simulink model "exampleModel_bus_axi_w_4ptavg"  (R2017b)
settings: Solver=VariableStepAuto  StartTime=0.0  StopTime=10e-5  RelTol=1e-3
PreLoadFcn:
  | setup
values from neighbouring files (symbols this model uses):
  axiClk = 156.25e6    (= 156250000)    [setup.m]    (also in setup_exampleModel_bus_axi_simulink.m; setup_exampleModel_bus_axi_simulink_lcls2.m; setup_lcls2_pcav.m; sysgen_signal.m)
  cav1p1_addr = 204    [setup_exampleModel_bus_axi_simulink.m]    (also in setup_exampleModel_bus_axi_simulink_lcls2.m; setup_lcls2_pcav.m; sysgen_signal.m)
  cav1p2_addr = cav1p1_addr * 2    (= 408)    [setup_exampleModel_bus_axi_simulink.m]    (also in setup_exampleModel_bus_axi_simulink_lcls2.m; setup_lcls2_pcav.m; sysgen_signal.m)
  cav2p1_addr = cav1p1_addr * 3    (= 612)    [setup_exampleModel_bus_axi_simulink.m]    (also in setup_exampleModel_bus_axi_simulink_lcls2.m; setup_lcls2_pcav.m; sysgen_signal.m)
  cav2p2_addr = cav1p1_addr * 4    (= 816)    [setup_exampleModel_bus_axi_simulink.m]    (also in setup_exampleModel_bus_axi_simulink_lcls2.m; setup_lcls2_pcav.m; sysgen_signal.m)
  Fadc = Fs/interleavedChannels    (= 29750000)    [setup.m]    (also in setup_exampleModel_bus_axi_simulink.m = 357000000; setup_exampleModel_bus_axi_simulink_lcls2.m = 351000000; setup_lcls2_pcav.m = 357000000; sysgen_signal.m = 357000000)
  fir_lpf = fir1(15, w_lpf)    [setup_exampleModel_bus_axi_simulink.m]    (also in setup_exampleModel_bus_axi_simulink_lcls2.m; setup_lcls2_pcav.m)
  Fproc = 204e6    (= 204000000)    [setup_exampleModel_bus_axi_simulink.m]    (also in setup_exampleModel_bus_axi_simulink_lcls2.m = 200571400; setup_lcls2_pcav.m; sysgen_signal.m)
  Fsig = Fproc/12    (= 17000000)    [setup_exampleModel_bus_axi_simulink.m]    (also in setup_exampleModel_bus_axi_simulink_lcls2.m = 16714283.3333; setup_lcls2_pcav.m)
  Tadc = 1/fadc    (= 2.80112044818e-09)    [cavity_signal.m]    (also in setup_exampleModel_bus_axi_simulink.m; setup_exampleModel_bus_axi_simulink_lcls2.m = 2.849002849e-09; setup_lcls2_pcav.m; setup_pcav_simulink.m)
undefined symbols (not defined in the file or in its folder): AXI4, Lite
libraries: xbsIndex_r4 x2870, llrf_lib x10, simulink x3
(part 2 of 15)

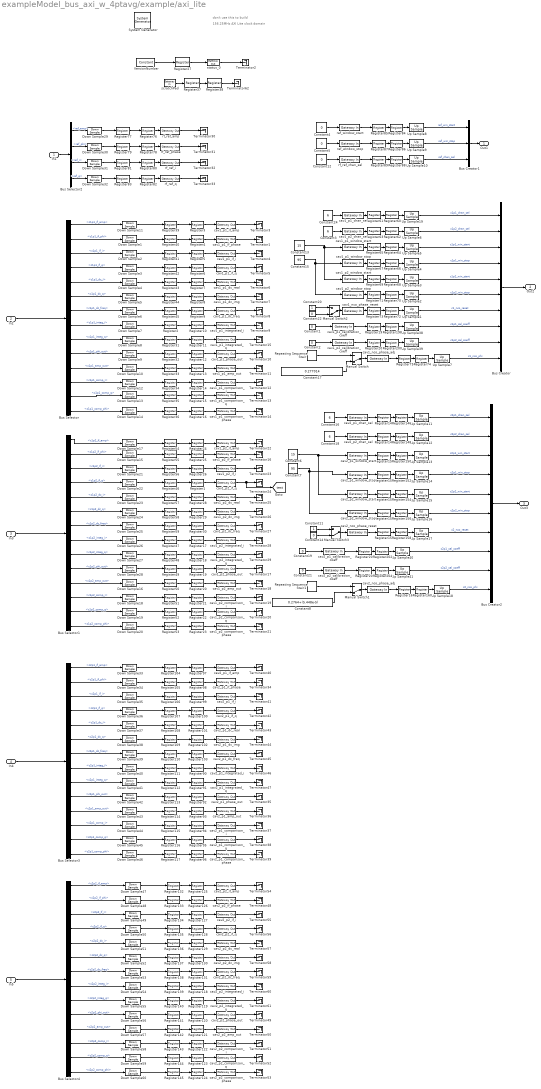
== system exampleModel_bus_axi_w_4ptavg/example/axi_lite ==
  note: don't use this to build
  note: 156.25MHz AXI Lite clock domain
  In1 : Inport
  In2 : Inport  Port=2
  In3 : Inport  Port=3
  In4 : Inport  Port=4
  In5 : Inport  Port=5
  " System Generator" : xbsIndex_r4/ System Generator  Tag=genX  xilinxfamily=kintexu  part=xcku040  speed=-2-e  package=ffva1156  synthesis_tool=Vivado  clock_wrapper=Clock Enables  directory=./netlist  proj_type=Vivado  Synth_file=Vivado Synthesis Defaults  Impl_file=Vivado Implementation Defaults  testbench=off  simulink_period=1/axiClk  sysclk_period=1e9/axiClk  dcm_input_clock_period=10  incr_netlist=off  trim_vbits=Everywhere in SubSystem  dbl_ovrd=According to Block Masks  core_generation=According to Block Masks  run_coregen=off  deprecated_control=off  eval_field=0  block_type=sysgen
  Bus Creator : BusCreator  Inputs=10
  Bus Creator1 : BusCreator  Inputs=3
  Bus Creator2 : BusCreator  Inputs=10
  Bus Selector : BusSelector  OutputSignals=c1p1_if_amp,c1p1_if_phi,c1p1_if_i,c1p1_if_q,c1p1_dc_i,c1p1_dc_q,c1p1_dc_freq,c1p1_integ_i,c1p1_integ_q,c1p1_phi_out,c1p1_amp_out,c1p1_comp_i,c1p1_comp_q,c1p1_comp_phi
  Bus Selector1 : BusSelector  OutputSignals=c1p2_if_amp,c1p2_if_phi,c1p2_if_i,c1p2_if_q,c1p2_dc_i,c1p2_dc_q,c1p2_dc_freq,c1p2_integ_i,c1p2_integ_q,c1p2_phi_out,c1p2_amp_out,c1p2_comp_i,c1p2_comp_q,c1p2_comp_phi
  Bus Selector2 : BusSelector  OutputSignals=ref_amp,ref_phi,ref_i,ref_q
  Bus Selector3 : BusSelector  OutputSignals=c2p1_if_amp,c2p1_if_phi,c2p1_if_i,c2p1_if_q,c2p1_dc_i,c2p1_dc_q,c2p1_dc_freq,c2p1_integ_i,c2p1_integ_q,c2p1_phi_out,c2p1_amp_out,c2p1_comp_i,c2p1_comp_q,c2p1_comp_phi
  Bus Selector4 : BusSelector  OutputSignals=c2p2_if_amp,c2p2_if_phi,c2p2_if_i,c2p2_if_q,c2p2_dc_i,c2p2_dc_q,c2p2_dc_freq,c2p2_integ_i,c2p2_integ_q,c2p2_phi_out,c2p2_amp_out,c2p2_comp_i,c2p2_comp_q,c2p2_comp_phi
  Constant{1..2,4..5,12,14,19,21..22} (9 alike) : Constant  Value=0  SampleTime=8/axiClk
  Constant11 : Constant  SampleTime=8/axiClk
  Constant13 : Constant  Value=15  SampleTime=8/axiClk
  Constant15 : Constant  Value=95  SampleTime=8/axiClk
  Constant{3,16,18,24} (4 alike) : Constant  Value=6  SampleTime=8/axiClk
  Constant17 : Constant  Value=0.277014  VectorParams1D=off  SampleTime=8/axiClk
  Constant20 : Constant  SampleTime=8/axiClk
  Constant6 : Constant  Value=15  SampleTime=8/axiClk
  Constant7 : Constant  Value=95  SampleTime=8/axiClk
  Constant8 : Constant  Value=0.2764+(5.448e-5)  VectorParams1D=off  SampleTime=8/axiClk
  Down Sample{1..60} (60 alike) : xbsIndex_r4/Down Sample  sample_ratio=8  sample_phase="Last Value of Frame  (most efficient)"  en=off  rst=off  latency=1  dbl_ovrd=off  block_type=dsamp
  Manual Switch{,1..3} (4 alike) : ManualSwitch  CurrentSetting=0
  Register{1..65,68..69,72..161,198..205} (165 alike) : xbsIndex_r4/Register  init=0  rst=off  en=off  dbl_ovrd=off  block_type=register
  Register{66..67,70..71} (4 alike) : xbsIndex_r4/Register  init=100  rst=off  en=off  dbl_ovrd=off  block_type=register
  Repeating Sequence Stair : simulink/Sources/Repeating Sequence Stair  OutValues=[0 (30/360) (45/360) (60/360) (75/360) (90/360) (8.2941/360)]  tsamp=0.5e-6  OutMin=[]  OutMax=[]  OutDataTypeStr=double  OutputDataTypeScalingMode=double  OutDataType=fixdt(0,8)  ConRadixGroup=Best Precision: Vector-wise  OutScaling=2^-12
  Repeating Sequence Stair1 : simulink/Sources/Repeating Sequence Stair  OutValues=[0 (30/360) (45/360) (60/360) (75/360) (90/360) (8.2941/360)]  tsamp=0.5e-6  OutMin=[]  OutMax=[]  OutDataTypeStr=double  OutputDataTypeScalingMode=double  OutDataType=fixdt(0,8)  ConRadixGroup=Best Precision: Vector-wise  OutScaling=2^-12
  Terminator{1..62} (62 alike) : Terminator
  Up Sample{1..19,38..41} (23 alike) : xbsIndex_r4/Up Sample  sample_ratio=8  copy_samples=on  en=off  latency=1  dbl_ovrd=off  block_type=usamp
  VersionNumber : xbsIndex_r4/Constant  const=7162020  gui_display_data_type=Fixed-point  arith_type=Unsigned  n_bits=32  bin_pt=0  preci_type=Single  exp_width=8  frac_width=24  explicit_period=on  period=8/axiClk  equ=P=C  opselect=C  inp2=PCIN>>17  opr=+  inp1=P  carry=CIN  dbl_ovrd=off  block_type=constant
  cav1_nco_phase_adj : xbsIndex_r4/Gateway In  gui_display_data_type=Fixed-point  arith_type=Unsigned  n_bits=32  bin_pt=32  preci_type=Single  exp_width=8  frac_width=24  rows=1  columns=1  quantization="Round  (unbiased: +/- Inf)"  overflow=Saturate  period=8/axiClk  UseAsADC=off  ADCChannel='1'  interface=AXI4-Lite  automatic_assignment=off  address_offset=cav1p1_addr+hex2dec('4C')  intf_name=''  intf_description=''  default_value=0  timing_constraint=None  locs_specified=off  LOCs={}  io_standard={}  inherit_from_input=off  hdl_port=on  dbl_ovrd=off  block_type=gatewayin
  cav1_nco_phase_reset : xbsIndex_r4/Gateway In  gui_display_data_type=Fixed-point  arith_type=Unsigned  n_bits=1  bin_pt=0  preci_type=Single  exp_width=8  frac_width=24  rows=1  columns=1  quantization="Round  (unbiased: +/- Inf)"  overflow=Saturate  period=8/axiClk  UseAsADC=off  ADCChannel='1'  interface=AXI4-Lite  automatic_assignment=off  address_offset=cav1p1_addr+hex2dec('50')  intf_name=''  intf_description=''  default_value=0  timing_constraint=None  locs_specified=off  LOCs={}  io_standard={}  inherit_from_input=off  hdl_port=on  dbl_ovrd=off  block_type=gatewayin
  cav1_p1_amp_out : xbsIndex_r4/Gateway Out  inherit_from_input=off  hdl_port=on  rows=1  columns=1  UseAsDAC=off  DACChannel='1'  interface=AXI4-Lite  automatic_assignment=off  address_offset=cav1p1_addr+hex2dec('34')  intf_name=''  intf_description=''  timing_constraint=None  locs_specified=off  LOCs={}  io_standard={}  block_type=gatewayout
  cav1_p1_calibration_coeff : xbsIndex_r4/Gateway In  gui_display_data_type=Fixed-point  arith_type=Unsigned  n_bits=18  bin_pt=17  preci_type=Single  exp_width=8  frac_width=24  rows=1  columns=1  quantization="Round  (unbiased: +/- Inf)"  overflow=Saturate  period=8/axiClk  UseAsADC=off  ADCChannel='1'  interface=AXI4-Lite  automatic_assignment=off  address_offset=cav1p1_addr+hex2dec('48')  intf_name=''  intf_description=''  default_value=0  timing_constraint=None  locs_specified=off  LOCs={}  io_standard={}  inherit_from_input=off  hdl_port=on  dbl_ovrd=off  block_type=gatewayin
  cav1_p1_chan_sel : xbsIndex_r4/Gateway In  gui_display_data_type=Fixed-point  arith_type=Unsigned  n_bits=4  bin_pt=0  preci_type=Single  exp_width=8  frac_width=24  rows=1  columns=1  quantization="Round  (unbiased: +/- Inf)"  overflow=Saturate  period=8/axiClk  UseAsADC=off  ADCChannel='1'  interface=AXI4-Lite  automatic_assignment=off  address_offset=cav1p1_addr+hex2dec('10')  intf_name=''  intf_description=''  default_value=0  timing_constraint=None  locs_specified=off  LOCs={}  io_standard={}  inherit_from_input=off  hdl_port=on  dbl_ovrd=off  block_type=gatewayin
  cav1_p1_comparison_i : xbsIndex_r4/Gateway Out  inherit_from_input=off  hdl_port=on  rows=1  columns=1  UseAsDAC=off  DACChannel='1'  interface=AXI4-Lite  automatic_assignment=off  address_offset=cav1p1_addr+hex2dec('38')  intf_name=''  intf_description=''  timing_constraint=None  locs_specified=off  LOCs={}  io_standard={}  block_type=gatewayout
  cav1_p1_comparison_phase : xbsIndex_r4/Gateway Out  inherit_from_input=off  hdl_port=on  rows=1  columns=1  UseAsDAC=off  DACChannel='1'  interface=AXI4-Lite  automatic_assignment=off  address_offset=cav1p1_addr+hex2dec('40')  intf_name=''  intf_description=''  timing_constraint=None  locs_specified=off  LOCs={}  io_standard={}  block_type=gatewayout
  cav1_p1_comparison_q : xbsIndex_r4/Gateway Out  inherit_from_input=off  hdl_port=on  rows=1  columns=1  UseAsDAC=off  DACChannel='1'  interface=AXI4-Lite  automatic_assignment=off  address_offset=cav1p1_addr+hex2dec('3C')  intf_name=''  intf_description=''  timing_constraint=None  locs_specified=off  LOCs={}  io_standard={}  block_type=gatewayout
  cav1_p1_dc_freq : xbsIndex_r4/Gateway Out  inherit_from_input=off  hdl_port=on  rows=1  columns=1  UseAsDAC=off  DACChannel='1'  interface=AXI4-Lite  automatic_assignment=off  address_offset=cav1p1_addr+hex2dec('24')  intf_name=''  intf_description=''  timing_constraint=None  locs_specified=off  LOCs={}  io_standard={}  block_type=gatewayout
  cav1_p1_dc_img : xbsIndex_r4/Gateway Out  inherit_from_input=off  hdl_port=on  rows=1  columns=1  UseAsDAC=off  DACChannel='1'  interface=AXI4-Lite  automatic_assignment=off  address_offset=cav1p1_addr+hex2dec('18')  intf_name=''  intf_description=''  timing_constraint=None  locs_specified=off  LOCs={}  io_standard={}  block_type=gatewayout
  cav1_p1_dc_real : xbsIndex_r4/Gateway Out  inherit_from_input=off  hdl_port=on  rows=1  columns=1  UseAsDAC=off  DACChannel='1'  interface=AXI4-Lite  automatic_assignment=off  address_offset=cav1p1_addr+hex2dec('14')  intf_name=''  intf_description=''  timing_constraint=None  locs_specified=off  LOCs={}  io_standard={}  block_type=gatewayout
  cav1_p1_if_amp : xbsIndex_r4/Gateway Out  inherit_from_input=off  hdl_port=on  rows=1  columns=1  UseAsDAC=off  DACChannel='1'  interface=AXI4-Lite  automatic_assignment=off  address_offset=cav1p1_addr+hex2dec('00')  intf_name=''  intf_description=''  timing_constraint=None  locs_specified=off  LOCs={}  io_standard={}  block_type=gatewayout
  cav1_p1_if_i : xbsIndex_r4/Gateway Out  inherit_from_input=off  hdl_port=on  rows=1  columns=1  UseAsDAC=off  DACChannel='1'  interface=AXI4-Lite  automatic_assignment=off  address_offset=cav1p1_addr+hex2dec('8')  intf_name=''  intf_description=''  timing_constraint=None  locs_specified=off  LOCs={}  io_standard={}  block_type=gatewayout
  cav1_p1_if_phase : xbsIndex_r4/Gateway Out  inherit_from_input=off  hdl_port=on  rows=1  columns=1  UseAsDAC=off  DACChannel='1'  interface=AXI4-Lite  automatic_assignment=off  address_offset=cav1p1_addr+hex2dec('4')  intf_name=''  intf_description=''  timing_constraint=None  locs_specified=off  LOCs={}  io_standard={}  block_type=gatewayout
  cav1_p1_if_q : xbsIndex_r4/Gateway Out  inherit_from_input=off  hdl_port=on  rows=1  columns=1  UseAsDAC=off  DACChannel='1'  interface=AXI4-Lite  automatic_assignment=off  address_offset=cav1p1_addr+hex2dec('c')  intf_name=''  intf_description=''  timing_constraint=None  locs_specified=off  LOCs={}  io_standard={}  block_type=gatewayout
  cav1_p1_integrated_i : xbsIndex_r4/Gateway Out  inherit_from_input=off  hdl_port=on  rows=1  columns=1  UseAsDAC=off  DACChannel='1'  interface=AXI4-Lite  automatic_assignment=off  address_offset=cav1p1_addr+hex2dec('28')  intf_name=''  intf_description=''  timing_constraint=None  locs_specified=off  LOCs={}  io_standard={}  block_type=gatewayout
  cav1_p1_integrated_q : xbsIndex_r4/Gateway Out  inherit_from_input=off  hdl_port=on  rows=1  columns=1  UseAsDAC=off  DACChannel='1'  interface=AXI4-Lite  automatic_assignment=off  address_offset=cav1p1_addr+hex2dec('2c')  intf_name=''  intf_description=''  timing_constraint=None  locs_specified=off  LOCs={}  io_standard={}  block_type=gatewayout
  cav1_p1_phase_out : xbsIndex_r4/Gateway Out  inherit_from_input=off  hdl_port=on  rows=1  columns=1  UseAsDAC=off  DACChannel='1'  interface=AXI4-Lite  automatic_assignment=off  address_offset=cav1p1_addr+hex2dec('30')  intf_name=''  intf_description=''  timing_constraint=None  locs_specified=off  LOCs={}  io_standard={}  block_type=gatewayout
  cav1_p1_window_start : xbsIndex_r4/Gateway In  gui_display_data_type=Fixed-point  arith_type=Unsigned  n_bits=16  bin_pt=0  preci_type=Single  exp_width=8  frac_width=24  rows=1  columns=1  quantization="Round  (unbiased: +/- Inf)"  overflow=Saturate  period=8/axiClk  UseAsADC=off  ADCChannel='1'  interface=AXI4-Lite  automatic_assignment=off  address_offset=cav1p1_addr+hex2dec('1C')  intf_name=''  intf_description=''  default_value=0  timing_constraint=None  locs_specified=off  LOCs={}  io_standard={}  inherit_from_input=off  hdl_port=on  dbl_ovrd=off  block_type=gatewayin
  cav1_p1_window_stop : xbsIndex_r4/Gateway In  gui_display_data_type=Fixed-point  arith_type=Unsigned  n_bits=16  bin_pt=0  preci_type=Single  exp_width=8  frac_width=24  rows=1  columns=1  quantization="Round  (unbiased: +/- Inf)"  overflow=Saturate  period=8/axiClk  UseAsADC=off  ADCChannel='1'  interface=AXI4-Lite  automatic_assignment=off  address_offset=cav1p1_addr+hex2dec('20')  intf_name=''  intf_description=''  default_value=100  timing_constraint=None  locs_specified=off  LOCs={}  io_standard={}  inherit_from_input=off  hdl_port=on  dbl_ovrd=off  block_type=gatewayin
  cav1_p2_amp_out : xbsIndex_r4/Gateway Out  inherit_from_input=off  hdl_port=on  rows=1  columns=1  UseAsDAC=off  DACChannel='1'  interface=AXI4-Lite  automatic_assignment=off  address_offset=cav1p2_addr+hex2dec('34')  intf_name=''  intf_description=''  timing_constraint=None  locs_specified=off  LOCs={}  io_standard={}  block_type=gatewayout
  cav1_p2_calibration_coeff : xbsIndex_r4/Gateway In  gui_display_data_type=Fixed-point  arith_type=Unsigned  n_bits=18  bin_pt=17  preci_type=Single  exp_width=8  frac_width=24  rows=1  columns=1  quantization="Round  (unbiased: +/- Inf)"  overflow=Saturate  period=8/axiClk  UseAsADC=off  ADCChannel='1'  interface=AXI4-Lite  automatic_assignment=off  address_offset=cav1p2_addr+hex2dec('48')  intf_name=''  intf_description=''  default_value=0  timing_constraint=None  locs_specified=off  LOCs={}  io_standard={}  inherit_from_input=off  hdl_port=on  dbl_ovrd=off  block_type=gatewayin
  cav1_p2_chan_sel : xbsIndex_r4/Gateway In  gui_display_data_type=Fixed-point  arith_type=Unsigned  n_bits=4  bin_pt=0  preci_type=Single  exp_width=8  frac_width=24  rows=1  columns=1  quantization="Round  (unbiased: +/- Inf)"  overflow=Saturate  period=8/axiClk  UseAsADC=off  ADCChannel='1'  interface=AXI4-Lite  automatic_assignment=off  address_offset=cav1p2_addr+hex2dec('10')  intf_name=''  intf_description=''  default_value=0  timing_constraint=None  locs_specified=off  LOCs={}  io_standard={}  inherit_from_input=off  hdl_port=on  dbl_ovrd=off  block_type=gatewayin
  cav1_p2_comparison_i : xbsIndex_r4/Gateway Out  inherit_from_input=off  hdl_port=on  rows=1  columns=1  UseAsDAC=off  DACChannel='1'  interface=AXI4-Lite  automatic_assignment=off  address_offset=cav1p2_addr+hex2dec('38')  intf_name=''  intf_description=''  timing_constraint=None  locs_specified=off  LOCs={}  io_standard={}  block_type=gatewayout
  cav1_p2_comparison_phase : xbsIndex_r4/Gateway Out  inherit_from_input=off  hdl_port=on  rows=1  columns=1  UseAsDAC=off  DACChannel='1'  interface=AXI4-Lite  automatic_assignment=off  address_offset=cav1p2_addr+hex2dec('40')  intf_name=''  intf_description=''  timing_constraint=None  locs_specified=off  LOCs={}  io_standard={}  block_type=gatewayout
  cav1_p2_comparison_q : xbsIndex_r4/Gateway Out  inherit_from_input=off  hdl_port=on  rows=1  columns=1  UseAsDAC=off  DACChannel='1'  interface=AXI4-Lite  automatic_assignment=off  address_offset=cav1p2_addr+hex2dec('3c')  intf_name=''  intf_description=''  timing_constraint=None  locs_specified=off  LOCs={}  io_standard={}  block_type=gatewayout
  cav1_p2_dc_freq : xbsIndex_r4/Gateway Out  inherit_from_input=off  hdl_port=on  rows=1  columns=1  UseAsDAC=off  DACChannel='1'  interface=AXI4-Lite  automatic_assignment=off  address_offset=cav1p2_addr+hex2dec('24')  intf_name=''  intf_description=''  timing_constraint=None  locs_specified=off  LOCs={}  io_standard={}  block_type=gatewayout
  cav1_p2_dc_img : xbsIndex_r4/Gateway Out  inherit_from_input=off  hdl_port=on  rows=1  columns=1  UseAsDAC=off  DACChannel='1'  interface=AXI4-Lite  automatic_assignment=off  address_offset=cav1p2_addr+hex2dec('18')  intf_name=''  intf_description=''  timing_constraint=None  locs_specified=off  LOCs={}  io_standard={}  block_type=gatewayout
  cav1_p2_dc_real : xbsIndex_r4/Gateway Out  inherit_from_input=off  hdl_port=on  rows=1  columns=1  UseAsDAC=off  DACChannel='1'  interface=AXI4-Lite  automatic_assignment=off  address_offset=cav1p2_addr+hex2dec('14')  intf_name=''  intf_description=''  timing_constraint=None  locs_specified=off  LOCs={}  io_standard={}  block_type=gatewayout
  cav1_p2_if_amp : xbsIndex_r4/Gateway Out  inherit_from_input=off  hdl_port=on  rows=1  columns=1  UseAsDAC=off  DACChannel='1'  interface=AXI4-Lite  automatic_assignment=off  address_offset=cav1p2_addr+hex2dec('00')  intf_name=''  intf_description=''  timing_constraint=None  locs_specified=off  LOCs={}  io_standard={}  block_type=gatewayout
  "cav1_p2_if_i " : xbsIndex_r4/Gateway Out  inherit_from_input=off  hdl_port=on  rows=1  columns=1  UseAsDAC=off  DACChannel='1'  interface=AXI4-Lite  automatic_assignment=off  address_offset=cav1p2_addr+hex2dec('08')  intf_name=''  intf_description=''  timing_constraint=None  locs_specified=off  LOCs={}  io_standard={}  block_type=gatewayout
  cav1_p2_if_phase : xbsIndex_r4/Gateway Out  inherit_from_input=off  hdl_port=on  rows=1  columns=1  UseAsDAC=off  DACChannel='1'  interface=AXI4-Lite  automatic_assignment=off  address_offset=cav1p2_addr+hex2dec('04')  intf_name=''  intf_description=''  timing_constraint=None  locs_specified=off  LOCs={}  io_standard={}  block_type=gatewayout
  cav1_p2_if_q : xbsIndex_r4/Gateway Out  inherit_from_input=off  hdl_port=on  rows=1  columns=1  UseAsDAC=off  DACChannel='1'  interface=AXI4-Lite  automatic_assignment=off  address_offset=cav1p2_addr+hex2dec('0C')  intf_name=''  intf_description=''  timing_constraint=None  locs_specified=off  LOCs={}  io_standard={}  block_type=gatewayout
  cav1_p2_integrated_i : xbsIndex_r4/Gateway Out  inherit_from_input=off  hdl_port=on  rows=1  columns=1  UseAsDAC=off  DACChannel='1'  interface=AXI4-Lite  automatic_assignment=off  address_offset=cav1p2_addr+hex2dec('28')  intf_name=''  intf_description=''  timing_constraint=None  locs_specified=off  LOCs={}  io_standard={}  block_type=gatewayout
  cav1_p2_integrated_q : xbsIndex_r4/Gateway Out  inherit_from_input=off  hdl_port=on  rows=1  columns=1  UseAsDAC=off  DACChannel='1'  interface=AXI4-Lite  automatic_assignment=off  address_offset=cav1p2_addr+hex2dec('2c')  intf_name=''  intf_description=''  timing_constraint=None  locs_specified=off  LOCs={}  io_standard={}  block_type=gatewayout
  cav1_p2_phase_out : xbsIndex_r4/Gateway Out  inherit_from_input=off  hdl_port=on  rows=1  columns=1  UseAsDAC=off  DACChannel='1'  interface=AXI4-Lite  automatic_assignment=off  address_offset=cav1p2_addr+hex2dec('30')  intf_name=''  intf_description=''  timing_constraint=None  locs_specified=off  LOCs={}  io_standard={}  block_type=gatewayout
  cav1_p2_window_start : xbsIndex_r4/Gateway In  gui_display_data_type=Fixed-point  arith_type=Unsigned  n_bits=16  bin_pt=0  preci_type=Single  exp_width=8  frac_width=24  rows=1  columns=1  quantization="Round  (unbiased: +/- Inf)"  overflow=Saturate  period=8/axiClk  UseAsADC=off  ADCChannel='1'  interface=AXI4-Lite  automatic_assignment=off  address_offset=cav1p2_addr+hex2dec('1c')  intf_name=''  intf_description=''  default_value=0  timing_constraint=None  locs_specified=off  LOCs={}  io_standard={}  inherit_from_input=off  hdl_port=on  dbl_ovrd=off  block_type=gatewayin
  cav1_p2_window_stop : xbsIndex_r4/Gateway In  gui_display_data_type=Fixed-point  arith_type=Unsigned  n_bits=16  bin_pt=0  preci_type=Single  exp_width=8  frac_width=24  rows=1  columns=1  quantization="Round  (unbiased: +/- Inf)"  overflow=Saturate  period=8/axiClk  UseAsADC=off  ADCChannel='1'  interface=AXI4-Lite  automatic_assignment=off  address_offset=cav1p2_addr+hex2dec('20')  intf_name=''  intf_description=''  default_value=100  timing_constraint=None  locs_specified=off  LOCs={}  io_standard={}  inherit_from_input=off  hdl_port=on  dbl_ovrd=off  block_type=gatewayin
  cav2_nco_phase_adj : xbsIndex_r4/Gateway In  gui_display_data_type=Fixed-point  arith_type=Unsigned  n_bits=32  bin_pt=32  preci_type=Single  exp_width=8  frac_width=24  rows=1  columns=1  quantization="Round  (unbiased: +/- Inf)"  overflow=Saturate  period=8/axiClk  UseAsADC=off  ADCChannel='1'  interface=AXI4-Lite  automatic_assignment=off  address_offset=cav2p1_addr+hex2dec('4c')  intf_name=''  intf_description=''  default_value=0  timing_constraint=None  locs_specified=off  LOCs={}  io_standard={}  inherit_from_input=off  hdl_port=on  dbl_ovrd=off  block_type=gatewayin
  cav2_nco_phase_reset : xbsIndex_r4/Gateway In  gui_display_data_type=Fixed-point  arith_type=Unsigned  n_bits=1  bin_pt=0  preci_type=Single  exp_width=8  frac_width=24  rows=1  columns=1  quantization="Round  (unbiased: +/- Inf)"  overflow=Saturate  period=8/axiClk  UseAsADC=off  ADCChannel='1'  interface=AXI4-Lite  automatic_assignment=off  address_offset=cav2p1_addr+hex2dec('50')  intf_name=''  intf_description=''  default_value=0  timing_constraint=None  locs_specified=off  LOCs={}  io_standard={}  inherit_from_input=off  hdl_port=on  dbl_ovrd=off  block_type=gatewayin
  cav2_p1_amp_out : xbsIndex_r4/Gateway Out  inherit_from_input=off  hdl_port=on  rows=1  columns=1  UseAsDAC=off  DACChannel='1'  interface=AXI4-Lite  automatic_assignment=off  address_offset=cav2p1_addr+hex2dec('34')  intf_name=''  intf_description=''  timing_constraint=None  locs_specified=off  LOCs={}  io_standard={}  block_type=gatewayout
  cav2_p1_calibration_coeff : xbsIndex_r4/Gateway In  gui_display_data_type=Fixed-point  arith_type=Unsigned  n_bits=18  bin_pt=17  preci_type=Single  exp_width=8  frac_width=24  rows=1  columns=1  quantization="Round  (unbiased: +/- Inf)"  overflow=Saturate  period=8/axiClk  UseAsADC=off  ADCChannel='1'  interface=AXI4-Lite  automatic_assignment=off  address_offset=cav2p1_addr+hex2dec('48')  intf_name=''  intf_description=''  default_value=0  timing_constraint=None  locs_specified=off  LOCs={}  io_standard={}  inherit_from_input=off  hdl_port=on  dbl_ovrd=off  block_type=gatewayin
  cav2_p1_chan_sel : xbsIndex_r4/Gateway In  gui_display_data_type=Fixed-point  arith_type=Unsigned  n_bits=4  bin_pt=0  preci_type=Single  exp_width=8  frac_width=24  rows=1  columns=1  quantization="Round  (unbiased: +/- Inf)"  overflow=Saturate  period=8/axiClk  UseAsADC=off  ADCChannel='1'  interface=AXI4-Lite  automatic_assignment=off  address_offset=cav2p1_addr+hex2dec('10')  intf_name=''  intf_description=''  default_value=0  timing_constraint=None  locs_specified=off  LOCs={}  io_standard={}  inherit_from_input=off  hdl_port=on  dbl_ovrd=off  block_type=gatewayin
  cav2_p1_comparison_i : xbsIndex_r4/Gateway Out  inherit_from_input=off  hdl_port=on  rows=1  columns=1  UseAsDAC=off  DACChannel='1'  interface=AXI4-Lite  automatic_assignment=off  address_offset=cav2p1_addr+hex2dec('38')  intf_name=''  intf_description=''  timing_constraint=None  locs_specified=off  LOCs={}  io_standard={}  block_type=gatewayout
  cav2_p1_comparison_phase : xbsIndex_r4/Gateway Out  inherit_from_input=off  hdl_port=on  rows=1  columns=1  UseAsDAC=off  DACChannel='1'  interface=AXI4-Lite  automatic_assignment=off  address_offset=cav2p1_addr+hex2dec('40')  intf_name=''  intf_description=''  timing_constraint=None  locs_specified=off  LOCs={}  io_standard={}  block_type=gatewayout
  cav2_p1_comparison_q : xbsIndex_r4/Gateway Out  inherit_from_input=off  hdl_port=on  rows=1  columns=1  UseAsDAC=off  DACChannel='1'  interface=AXI4-Lite  automatic_assignment=off  address_offset=cav2p1_addr+hex2dec('3c')  intf_name=''  intf_description=''  timing_constraint=None  locs_specified=off  LOCs={}  io_standard={}  block_type=gatewayout
  cav2_p1_dc_freq : xbsIndex_r4/Gateway Out  inherit_from_input=off  hdl_port=on  rows=1  columns=1  UseAsDAC=off  DACChannel='1'  interface=AXI4-Lite  automatic_assignment=off  address_offset=cav2p1_addr+hex2dec('24')  intf_name=''  intf_description=''  timing_constraint=None  locs_specified=off  LOCs={}  io_standard={}  block_type=gatewayout
  cav2_p1_dc_img : xbsIndex_r4/Gateway Out  inherit_from_input=off  hdl_port=on  rows=1  columns=1  UseAsDAC=off  DACChannel='1'  interface=AXI4-Lite  automatic_assignment=off  address_offset=cav2p1_addr+hex2dec('18')  intf_name=''  intf_description=''  timing_constraint=None  locs_specified=off  LOCs={}  io_standard={}  block_type=gatewayout
  cav2_p1_dc_real : xbsIndex_r4/Gateway Out  inherit_from_input=off  hdl_port=on  rows=1  columns=1  UseAsDAC=off  DACChannel='1'  interface=AXI4-Lite  automatic_assignment=off  address_offset=cav2p1_addr+hex2dec('14')  intf_name=''  intf_description=''  timing_constraint=None  locs_specified=off  LOCs={}  io_standard={}  block_type=gatewayout
  cav2_p1_if_amp : xbsIndex_r4/Gateway Out  inherit_from_input=off  hdl_port=on  rows=1  columns=1  UseAsDAC=off  DACChannel='1'  interface=AXI4-Lite  automatic_assignment=off  address_offset=cav2p1_addr+hex2dec('0')  intf_name=''  intf_description=''  timing_constraint=None  locs_specified=off  LOCs={}  io_standard={}  block_type=gatewayout
  cav2_p1_if_i : xbsIndex_r4/Gateway Out  inherit_from_input=off  hdl_port=on  rows=1  columns=1  UseAsDAC=off  DACChannel='1'  interface=AXI4-Lite  automatic_assignment=off  address_offset=cav2p1_addr+hex2dec('8')  intf_name=''  intf_description=''  timing_constraint=None  locs_specified=off  LOCs={}  io_standard={}  block_type=gatewayout
  cav2_p1_if_phase : xbsIndex_r4/Gateway Out  inherit_from_input=off  hdl_port=on  rows=1  columns=1  UseAsDAC=off  DACChannel='1'  interface=AXI4-Lite  automatic_assignment=off  address_offset=cav2p1_addr+hex2dec('4')  intf_name=''  intf_description=''  timing_constraint=None  locs_specified=off  LOCs={}  io_standard={}  block_type=gatewayout
  cav2_p1_if_q : xbsIndex_r4/Gateway Out  inherit_from_input=off  hdl_port=on  rows=1  columns=1  UseAsDAC=off  DACChannel='1'  interface=AXI4-Lite  automatic_assignment=off  address_offset=cav2p1_addr+hex2dec('c')  intf_name=''  intf_description=''  timing_constraint=None  locs_specified=off  LOCs={}  io_standard={}  block_type=gatewayout
  cav2_p1_integrated_i : xbsIndex_r4/Gateway Out  inherit_from_input=off  hdl_port=on  rows=1  columns=1  UseAsDAC=off  DACChannel='1'  interface=AXI4-Lite  automatic_assignment=off  address_offset=cav2p1_addr+hex2dec('28')  intf_name=''  intf_description=''  timing_constraint=None  locs_specified=off  LOCs={}  io_standard={}  block_type=gatewayout
  cav2_p1_integrated_q : xbsIndex_r4/Gateway Out  inherit_from_input=off  hdl_port=on  rows=1  columns=1  UseAsDAC=off  DACChannel='1'  interface=AXI4-Lite  automatic_assignment=off  address_offset=cav2p1_addr+hex2dec('2c')  intf_name=''  intf_description=''  timing_constraint=None  locs_specified=off  LOCs={}  io_standard={}  block_type=gatewayout
  cav2_p1_phase_out : xbsIndex_r4/Gateway Out  inherit_from_input=off  hdl_port=on  rows=1  columns=1  UseAsDAC=off  DACChannel='1'  interface=AXI4-Lite  automatic_assignment=off  address_offset=cav2p1_addr+hex2dec('30')  intf_name=''  intf_description=''  timing_constraint=None  locs_specified=off  LOCs={}  io_standard={}  block_type=gatewayout
  cav2_p1_window_start : xbsIndex_r4/Gateway In  gui_display_data_type=Fixed-point  arith_type=Unsigned  n_bits=16  bin_pt=0  preci_type=Single  exp_width=8  frac_width=24  rows=1  columns=1  quantization="Round  (unbiased: +/- Inf)"  overflow=Saturate  period=8/axiClk  UseAsADC=off  ADCChannel='1'  interface=AXI4-Lite  automatic_assignment=off  address_offset=cav2p1_addr+hex2dec('1c')  intf_name=''  intf_description=''  default_value=0  timing_constraint=None  locs_specified=off  LOCs={}  io_standard={}  inherit_from_input=off  hdl_port=on  dbl_ovrd=off  block_type=gatewayin
  cav2_p1_window_stop : xbsIndex_r4/Gateway In  gui_display_data_type=Fixed-point  arith_type=Unsigned  n_bits=16  bin_pt=0  preci_type=Single  exp_width=8  frac_width=24  rows=1  columns=1  quantization="Round  (unbiased: +/- Inf)"  overflow=Saturate  period=8/axiClk  UseAsADC=off  ADCChannel='1'  interface=AXI4-Lite  automatic_assignment=off  address_offset=cav2p1_addr+hex2dec('20')  intf_name=''  intf_description=''  default_value=0  timing_constraint=None  locs_specified=off  LOCs={}  io_standard={}  inherit_from_input=off  hdl_port=on  dbl_ovrd=off  block_type=gatewayin
  cav2_p2_amp_out : xbsIndex_r4/Gateway Out  inherit_from_input=off  hdl_port=on  rows=1  columns=1  UseAsDAC=off  DACChannel='1'  interface=AXI4-Lite  automatic_assignment=off  address_offset=cav2p2_addr+hex2dec('34')  intf_name=''  intf_description=''  timing_constraint=None  locs_specified=off  LOCs={}  io_standard={}  block_type=gatewayout
  cav2_p2_calibration_coeff : xbsIndex_r4/Gateway In  gui_display_data_type=Fixed-point  arith_type=Unsigned  n_bits=18  bin_pt=17  preci_type=Single  exp_width=8  frac_width=24  rows=1  columns=1  quantization="Round  (unbiased: +/- Inf)"  overflow=Saturate  period=8/axiClk  UseAsADC=off  ADCChannel='1'  interface=AXI4-Lite  automatic_assignment=off  address_offset=cav2p2_addr+hex2dec('48')  intf_name=''  intf_description=''  default_value=0  timing_constraint=None  locs_specified=off  LOCs={}  io_standard={}  inherit_from_input=off  hdl_port=on  dbl_ovrd=off  block_type=gatewayin
  cav2_p2_chan_sel : xbsIndex_r4/Gateway In  gui_display_data_type=Fixed-point  arith_type=Unsigned  n_bits=4  bin_pt=0  preci_type=Single  exp_width=8  frac_width=24  rows=1  columns=1  quantization="Round  (unbiased: +/- Inf)"  overflow=Saturate  period=8/axiClk  UseAsADC=off  ADCChannel='1'  interface=AXI4-Lite  automatic_assignment=off  address_offset=cav2p2_addr+hex2dec('10')  intf_name=''  intf_description=''  default_value=0  timing_constraint=None  locs_specified=off  LOCs={}  io_standard={}  inherit_from_input=off  hdl_port=on  dbl_ovrd=off  block_type=gatewayin
  cav2_p2_comparison_i : xbsIndex_r4/Gateway Out  inherit_from_input=off  hdl_port=on  rows=1  columns=1  UseAsDAC=off  DACChannel='1'  interface=AXI4-Lite  automatic_assignment=off  address_offset=cav2p2_addr+hex2dec('38')  intf_name=''  intf_description=''  timing_constraint=None  locs_specified=off  LOCs={}  io_standard={}  block_type=gatewayout
  cav2_p2_comparison_phase : xbsIndex_r4/Gateway Out  inherit_from_input=off  hdl_port=on  rows=1  columns=1  UseAsDAC=off  DACChannel='1'  interface=AXI4-Lite  automatic_assignment=off  address_offset=cav2p2_addr+hex2dec('40')  intf_name=''  intf_description=''  timing_constraint=None  locs_specified=off  LOCs={}  io_standard={}  block_type=gatewayout
  cav2_p2_comparison_q : xbsIndex_r4/Gateway Out  inherit_from_input=off  hdl_port=on  rows=1  columns=1  UseAsDAC=off  DACChannel='1'  interface=AXI4-Lite  automatic_assignment=off  address_offset=cav2p2_addr+hex2dec('3c')  intf_name=''  intf_description=''  timing_constraint=None  locs_specified=off  LOCs={}  io_standard={}  block_type=gatewayout
  cav2_p2_dc_freq : xbsIndex_r4/Gateway Out  inherit_from_input=off  hdl_port=on  rows=1  columns=1  UseAsDAC=off  DACChannel='1'  interface=AXI4-Lite  automatic_assignment=off  address_offset=cav2p2_addr+hex2dec('24')  intf_name=''  intf_description=''  timing_constraint=None  locs_specified=off  LOCs={}  io_standard={}  block_type=gatewayout
  cav2_p2_dc_img : xbsIndex_r4/Gateway Out  inherit_from_input=off  hdl_port=on  rows=1  columns=1  UseAsDAC=off  DACChannel='1'  interface=AXI4-Lite  automatic_assignment=off  address_offset=cav2p2_addr+hex2dec('18')  intf_name=''  intf_description=''  timing_constraint=None  locs_specified=off  LOCs={}  io_standard={}  block_type=gatewayout
  cav2_p2_dc_real : xbsIndex_r4/Gateway Out  inherit_from_input=off  hdl_port=on  rows=1  columns=1  UseAsDAC=off  DACChannel='1'  interface=AXI4-Lite  automatic_assignment=off  address_offset=cav2p2_addr+hex2dec('14')  intf_name=''  intf_description=''  timing_constraint=None  locs_specified=off  LOCs={}  io_standard={}  block_type=gatewayout
  cav2_p2_if_amp : xbsIndex_r4/Gateway Out  inherit_from_input=off  hdl_port=on  rows=1  columns=1  UseAsDAC=off  DACChannel='1'  interface=AXI4-Lite  automatic_assignment=off  address_offset=cav2p2_addr+hex2dec('0')  intf_name=''  intf_description=''  timing_constraint=None  locs_specified=off  LOCs={}  io_standard={}  block_type=gatewayout
  "cav2_p2_if_i " : xbsIndex_r4/Gateway Out  inherit_from_input=off  hdl_port=on  rows=1  columns=1  UseAsDAC=off  DACChannel='1'  interface=AXI4-Lite  automatic_assignment=off  address_offset=cav2p2_addr+hex2dec('8')  intf_name=''  intf_description=''  timing_constraint=None  locs_specified=off  LOCs={}  io_standard={}  block_type=gatewayout
  cav2_p2_if_phase : xbsIndex_r4/Gateway Out  inherit_from_input=off  hdl_port=on  rows=1  columns=1  UseAsDAC=off  DACChannel='1'  interface=AXI4-Lite  automatic_assignment=off  address_offset=cav2p2_addr+hex2dec('4')  intf_name=''  intf_description=''  timing_constraint=None  locs_specified=off  LOCs={}  io_standard={}  block_type=gatewayout
  cav2_p2_if_q : xbsIndex_r4/Gateway Out  inherit_from_input=off  hdl_port=on  rows=1  columns=1  UseAsDAC=off  DACChannel='1'  interface=AXI4-Lite  automatic_assignment=off  address_offset=cav2p2_addr+hex2dec('c')  intf_name=''  intf_description=''  timing_constraint=None  locs_specified=off  LOCs={}  io_standard={}  block_type=gatewayout
  cav2_p2_integrated_i : xbsIndex_r4/Gateway Out  inherit_from_input=off  hdl_port=on  rows=1  columns=1  UseAsDAC=off  DACChannel='1'  interface=AXI4-Lite  automatic_assignment=off  address_offset=cav2p2_addr+hex2dec('28')  intf_name=''  intf_description=''  timing_constraint=None  locs_specified=off  LOCs={}  io_standard={}  block_type=gatewayout
  cav2_p2_integrated_q : xbsIndex_r4/Gateway Out  inherit_from_input=off  hdl_port=on  rows=1  columns=1  UseAsDAC=off  DACChannel='1'  interface=AXI4-Lite  automatic_assignment=off  address_offset=cav2p2_addr+hex2dec('2c')  intf_name=''  intf_description=''  timing_constraint=None  locs_specified=off  LOCs={}  io_standard={}  block_type=gatewayout
  cav2_p2_phase_out : xbsIndex_r4/Gateway Out  inherit_from_input=off  hdl_port=on  rows=1  columns=1  UseAsDAC=off  DACChannel='1'  interface=AXI4-Lite  automatic_assignment=off  address_offset=cav2p2_addr+hex2dec('30')  intf_name=''  intf_description=''  timing_constraint=None  locs_specified=off  LOCs={}  io_standard={}  block_type=gatewayout
  cav2_p2_window_start : xbsIndex_r4/Gateway In  gui_display_data_type=Fixed-point  arith_type=Unsigned  n_bits=16  bin_pt=0  preci_type=Single  exp_width=8  frac_width=24  rows=1  columns=1  quantization="Round  (unbiased: +/- Inf)"  overflow=Saturate  period=8/axiClk  UseAsADC=off  ADCChannel='1'  interface=AXI4-Lite  automatic_assignment=off  address_offset=cav2p2_addr+hex2dec('1c')  intf_name=''  intf_description=''  default_value=0  timing_constraint=None  locs_specified=off  LOCs={}  io_standard={}  inherit_from_input=off  hdl_port=on  dbl_ovrd=off  block_type=gatewayin
  cav2_p2_window_stop : xbsIndex_r4/Gateway In  gui_display_data_type=Fixed-point  arith_type=Unsigned  n_bits=16  bin_pt=0  preci_type=Single  exp_width=8  frac_width=24  rows=1  columns=1  quantization="Round  (unbiased: +/- Inf)"  overflow=Saturate  period=8/axiClk  UseAsADC=off  ADCChannel='1'  interface=AXI4-Lite  automatic_assignment=off  address_offset=cav2p2_addr+hex2dec('20')  intf_name=''  intf_description=''  default_value=0  timing_constraint=None  locs_specified=off  LOCs={}  io_standard={}  inherit_from_input=off  hdl_port=on  dbl_ovrd=off  block_type=gatewayin
  ref_window_start : xbsIndex_r4/Gateway In  gui_display_data_type=Fixed-point  arith_type=Unsigned  n_bits=16  bin_pt=0  preci_type=Single  exp_width=8  frac_width=24  rows=1  columns=1  quantization="Round  (unbiased: +/- Inf)"  overflow=Saturate  period=8/axiClk  UseAsADC=off  ADCChannel='1'  interface=AXI4-Lite  automatic_assignment=off  address_offset=hex2dec('14')  intf_name=''  intf_description=''  default_value=0  timing_constraint=None  locs_specified=off  LOCs={}  io_standard={}  inherit_from_input=off  hdl_port=on  dbl_ovrd=off  block_type=gatewayin
  ref_window_stop : xbsIndex_r4/Gateway In  gui_display_data_type=Fixed-point  arith_type=Unsigned  n_bits=16  bin_pt=0  preci_type=Single  exp_width=8  frac_width=24  rows=1  columns=1  quantization="Round  (unbiased: +/- Inf)"  overflow=Saturate  period=8/axiClk  UseAsADC=off  ADCChannel='1'  interface=AXI4-Lite  automatic_assignment=off  address_offset=hex2dec('18')  intf_name=''  intf_description=''  default_value=0  timing_constraint=None  locs_specified=off  LOCs={}  io_standard={}  inherit_from_input=off  hdl_port=on  dbl_ovrd=off  block_type=gatewayin
  rf_ref_amp : xbsIndex_r4/Gateway Out  inherit_from_input=off  hdl_port=on  rows=1  columns=1  UseAsDAC=off  DACChannel='1'  interface=AXI4-Lite  automatic_assignment=off  address_offset=hex2dec('00')  intf_name=''  intf_description=''  timing_constraint=None  locs_specified=off  LOCs={}  io_standard={}  block_type=gatewayout
  rf_ref_chan_sel : xbsIndex_r4/Gateway In  gui_display_data_type=Fixed-point  arith_type=Unsigned  n_bits=4  bin_pt=0  preci_type=Single  exp_width=8  frac_width=24  rows=1  columns=1  quantization="Round  (unbiased: +/- Inf)"  overflow=Saturate  period=8/axiClk  UseAsADC=off  ADCChannel='1'  interface=AXI4-Lite  automatic_assignment=off  address_offset=hex2dec('10')  intf_name=''  intf_description=''  default_value=0  timing_constraint=None  locs_specified=off  LOCs={}  io_standard={}  inherit_from_input=off  hdl_port=on  dbl_ovrd=off  block_type=gatewayin
  rf_ref_i : xbsIndex_r4/Gateway Out  inherit_from_input=off  hdl_port=on  rows=1  columns=1  UseAsDAC=off  DACChannel='1'  interface=AXI4-Lite  automatic_assignment=off  address_offset=hex2dec('08')  intf_name=''  intf_description=''  timing_constraint=None  locs_specified=off  LOCs={}  io_standard={}  block_type=gatewayout
  rf_ref_phase : xbsIndex_r4/Gateway Out  inherit_from_input=off  hdl_port=on  rows=1  columns=1  UseAsDAC=off  DACChannel='1'  interface=AXI4-Lite  automatic_assignment=off  address_offset=hex2dec('04')  intf_name=''  intf_description=''  timing_constraint=None  locs_specified=off  LOCs={}  io_standard={}  block_type=gatewayout
  rf_ref_q : xbsIndex_r4/Gateway Out  inherit_from_input=off  hdl_port=on  rows=1  columns=1  UseAsDAC=off  DACChannel='1'  interface=AXI4-Lite  automatic_assignment=off  address_offset=hex2dec('0C')  intf_name=''  intf_description=''  timing_constraint=None  locs_specified=off  LOCs={}  io_standard={}  block_type=gatewayout
  scratchPad : xbsIndex_r4/Gateway In  gui_display_data_type=Fixed-point  arith_type=Unsigned  n_bits=32  bin_pt=0  preci_type=Single  exp_width=8  frac_width=24  rows=1  columns=1  quantization="Round  (unbiased: +/- Inf)"  overflow=Saturate  period=8/axiClk  UseAsADC=off  ADCChannel='1'  interface=AXI4-Lite  automatic_assignment=off  address_offset=4092  intf_name=''  intf_description=''  default_value=0  timing_constraint=None  locs_specified=off  LOCs={}  io_standard={}  inherit_from_input=off  hdl_port=on  dbl_ovrd=off  block_type=gatewayin
  status_0 : xbsIndex_r4/Gateway Out  inherit_from_input=on  hdl_port=on  rows=1  columns=1  UseAsDAC=off  DACChannel='1'  interface=AXI4-Lite  automatic_assignment=off  address_offset=hex2dec('3f8')  intf_name=''  intf_description=''  timing_constraint=None  locs_specified=off  LOCs={}  io_standard={}  block_type=gatewayout
  Out1 : Outport
  Out2 : Outport  Port=2
  Out3 : Outport  Port=3
  tag scope: test=global
  wires:
  VersionNumber/1 -> Register27/1
  Register27/1 -> status_0/1
  status_0/1 -> Terminator2/1
  scratchPad/1 -> Register37/1
  Register37/1 -> Register38/1
  Bus Selector/14 -> Down Sample14/1  "<c1p1_comp_phi>"
  cav1_p1_comparison_phase/1 -> Terminator14/1
  Register3/1 -> cav1_p1_if_amp/1
  Register10/1 -> cav1_p1_integrated_i/1
  cav1_p1_comparison_q/1 -> Terminator13/1
  cav1_p1_comparison_i/1 -> Terminator12/1
  cav1_p1_phase_out/1 -> Terminator10/1
  Register6/1 -> cav1_p1_if_q/1
  cav1_p1_dc_img/1 -> Terminator7/1
  Register16/1 -> cav1_p1_comparison_phase/1
  Bus Selector/9 -> Down Sample8/1  "<c1p1_integ_q>"
  Bus Selector/5 -> Down Sample4/1  "<c1p1_dc_i>"
  Bus Selector/11 -> Down Sample10/1  "<c1p1_amp_out>"
  Register13/1 -> cav1_p1_amp_out/1
  Bus Selector/7 -> Down Sample6/1  "<c1p1_dc_freq>"
  Bus Selector/1 -> Down Sample11/1  "<c1p1_if_amp>"
  Bus Selector/2 -> Down Sample1/1  "<c1p1_if_phi>"
  cav1_p1_dc_freq/1 -> Terminator8/1
  Register15/1 -> cav1_p1_comparison_q/1
  Register5/1 -> cav1_p1_if_i/1
  cav1_p1_integrated_q/1 -> Terminator15/1
  Bus Selector/6 -> Down Sample5/1  "<c1p1_dc_q>"
  cav1_p1_integrated_i/1 -> Terminator9/1
  cav1_p1_if_amp/1 -> Terminator3/1
  cav1_p1_dc_real/1 -> Terminator6/1
  Register8/1 -> cav1_p1_dc_img/1
  Bus Selector/3 -> Down Sample2/1  "<c1p1_if_i>"
  Register7/1 -> cav1_p1_dc_real/1
  Register4/1 -> cav1_p1_if_phase/1
  Register14/1 -> cav1_p1_comparison_i/1
  Register9/1 -> cav1_p1_dc_freq/1
  Register12/1 -> cav1_p1_phase_out/1
  cav1_p1_amp_out/1 -> Terminator11/1
  Bus Selector/8 -> Down Sample7/1  "<c1p1_integ_i>"
  Register11/1 -> cav1_p1_integrated_q/1
  Bus Selector/4 -> Down Sample3/1  "<c1p1_if_q>"
  Bus Selector/12 -> Down Sample12/1  "<c1p1_comp_i>"
  cav1_p1_if_q/1 -> Terminator5/1
  cav1_p1_if_i/1 -> Terminator4/1
  cav1_p1_if_phase/1 -> Terminator1/1
  Bus Selector/13 -> Down Sample13/1  "<c1p1_comp_q>"
  Bus Selector/10 -> Down Sample9/1  "<c1p1_phi_out>"
  Down Sample11/1 -> Register39/1
  Down Sample1/1 -> Register40/1
  Down Sample2/1 -> Register41/1
  Down Sample3/1 -> Register42/1
  Down Sample4/1 -> Register43/1
  Down Sample5/1 -> Register44/1
  Down Sample6/1 -> Register45/1
  Down Sample7/1 -> Register2/1
  Down Sample8/1 -> Register31/1
  Down Sample9/1 -> Register32/1
  Down Sample10/1 -> Register33/1
  Down Sample12/1 -> Register34/1
  Down Sample13/1 -> Register35/1
  Down Sample14/1 -> Register36/1
  Down Sample22/1 -> Register46/1
  Down Sample19/1 -> Register52/1
  Down Sample26/1 -> Register47/1
  Register26/1 -> "cav1_p2_if_i "/1
  Down Sample20/1 -> Register53/1
  Down Sample17/1 -> Register54/1
  cav1_p2_dc_freq/1 -> Terminator27/1
  Down Sample15/1 -> Register55/1
  Down Sample23/1 -> Register57/1
  cav1_p2_amp_out/1 -> Terminator18/1
  cav1_p2_if_amp/1 -> Terminator22/1
  "cav1_p2_if_i "/1 -> Terminator23/1
  Register29/1 -> cav1_p2_dc_img/1
  Register22/1 -> cav1_p2_comparison_q/1
  Register23/1 -> cav1_p2_comparison_phase/1
  Register30/1 -> cav1_p2_dc_freq/1
  Register17/1 -> cav1_p2_integrated_i/1
  Down Sample28/1 -> Register49/1
  cav1_p2_if_q/1 -> [test], Terminator24/1
  Down Sample27/1 -> Register48/1
  Register25/1 -> cav1_p2_if_phase/1
  Register1/1 -> cav1_p2_if_q/1
  Down Sample21/1 -> Register56/1
  Register21/1 -> cav1_p2_comparison_i/1
  cav1_p2_dc_real/1 -> Terminator25/1
  cav1_p2_dc_img/1 -> Terminator26/1
  Down Sample24/1 -> Register58/1
  Down Sample18/1 -> Register51/1
  Register24/1 -> cav1_p2_if_amp/1
  cav1_p2_phase_out/1 -> Terminator17/1
  Down Sample25/1 -> Register59/1
  cav1_p2_integrated_q/1 -> Terminator29/1
  cav1_p2_comparison_q/1 -> Terminator20/1
  Down Sample16/1 -> Register50/1
  cav1_p2_comparison_phase/1 -> Terminator21/1
  cav1_p2_if_phase/1 -> Terminator16/1
  Register20/1 -> cav1_p2_amp_out/1
  cav1_p2_comparison_i/1 -> Terminator19/1
  Register18/1 -> cav1_p2_integrated_q/1
  Register19/1 -> cav1_p2_phase_out/1
  cav1_p2_integrated_i/1 -> Terminator28/1
  Register28/1 -> cav1_p2_dc_real/1
  Bus Selector1/9 -> Down Sample27/1  "<c1p2_integ_q>"
  Bus Selector1/8 -> Down Sample26/1  "<c1p2_integ_i>"
  Bus Selector1/4 -> Down Sample22/1  "<c1p2_if_q>"
  Bus Selector1/14 -> Down Sample20/1  "<c1p2_comp_phi>"
  Bus Selector1/1 -> Down Sample17/1  "<c1p2_if_amp>"
  Bus Selector1/5 -> Down Sample23/1  "<c1p2_dc_i>"
  Bus Selector1/12 -> Down Sample18/1  "<c1p2_comp_i>"
  Bus Selector1/7 -> Down Sample25/1  "<c1p2_dc_freq>"
  Bus Selector1/3 -> Down Sample21/1  "<c1p2_if_i>"
  Bus Selector1/11 -> Down Sample16/1  "<c1p2_amp_out>"
  Bus Selector1/2 -> Down Sample15/1  "<c1p2_if_phi>"
  Bus Selector1/6 -> Down Sample24/1  "<c1p2_dc_q>"
  Bus Selector1/10 -> Down Sample28/1  "<c1p2_phi_out>"
  Bus Selector1/13 -> Down Sample19/1  "<c1p2_comp_q>"
  Constant22/1 -> Manual Switch2/2
  Manual Switch/1 -> cav1_nco_phase_adj/1
  Constant17/1 -> Manual Switch/2
  Constant20/1 -> Manual Switch2/1
  Constant24/1 -> cav1_p1_chan_sel/1
  Constant15/1 -> cav1_p2_window_stop/1, cav1_p1_window_stop/1
  Constant13/1 -> cav1_p2_window_start/1, cav1_p1_window_start/1
  Repeating Sequence Stair/1 -> Manual Switch/1
  Manual Switch2/1 -> cav1_nco_phase_reset/1
  Register43/1 -> Register7/1
  Register36/1 -> Register16/1
  Register41/1 -> Register5/1
  Register31/1 -> Register11/1
  Register2/1 -> Register10/1
  Register45/1 -> Register9/1
  Register33/1 -> Register13/1
  Register32/1 -> Register12/1
  Register34/1 -> Register14/1
  Register35/1 -> Register15/1
  Register44/1 -> Register8/1
  Register40/1 -> Register4/1
  Register39/1 -> Register3/1
  Register42/1 -> Register6/1
  Register51/1 -> Register21/1
  Register48/1 -> Register18/1
  Register58/1 -> Register29/1
  Register56/1 -> Register26/1
  Register57/1 -> Register28/1
  Register54/1 -> Register24/1
  Register47/1 -> Register17/1
  Register46/1 -> Register1/1
  Register49/1 -> Register19/1
  Register50/1 -> Register20/1
  Register59/1 -> Register30/1
  Register55/1 -> Register25/1
  Register53/1 -> Register23/1
  Register52/1 -> Register22/1
  Constant3/1 -> cav1_p2_chan_sel/1
  Register61/1 -> Register60/1
  Register60/1 -> Up Sample19/1
  cav1_p1_chan_sel/1 -> Register61/1
  Up Sample19/1 -> Bus Creator/1  "c1p1_chan_sel"
  Register62/1 -> Up Sample6/1
  Register63/1 -> Register62/1
  Up Sample6/1 -> Bus Creator/2  "c1p2_chan_sel"
  cav1_p2_chan_sel/1 -> Register63/1
  Register64/1 -> Up Sample5/1
  Register65/1 -> Register64/1
  cav1_p1_window_start/1 -> Register65/1
  Up Sample5/1 -> Bus Creator/3  "c1p1_win_start"
  Register66/1 -> Up Sample4/1
  Register67/1 -> Register66/1
  Up Sample4/1 -> Bus Creator/4  "c1p1_win_stop"
  cav1_p1_window_stop/1 -> Register67/1
  Register68/1 -> Up Sample3/1
  Register69/1 -> Register68/1
  Up Sample3/1 -> Bus Creator/5  "c1p2_win_start"
  cav1_p2_window_start/1 -> Register69/1
  Register70/1 -> Up Sample2/1
  Register71/1 -> Register70/1
  Up Sample2/1 -> Bus Creator/6  "c1p2_win_stop"
  cav1_p2_window_stop/1 -> Register71/1
  Register72/1 -> Up Sample1/1
  Register73/1 -> Register72/1
  cav1_nco_phase_reset/1 -> Register73/1
  Up Sample1/1 -> Bus Creator/7  "c1_nco_reset"
  Register74/1 -> Up Sample7/1
  Register75/1 -> Register74/1
  cav1_nco_phase_adj/1 -> Register75/1
  Up Sample7/1 -> Bus Creator/10  "c1_nco_phi"
  In2/1 -> Bus Selector/1
  In3/1 -> Bus Selector1/1
  Bus Creator/1 -> Out2/1
  Constant4/1 -> ref_window_start/1
  ref_window_start/1 -> Register85/1
  ref_window_stop/1 -> Register87/1
  rf_ref_chan_sel/1 -> Register89/1
  Constant5/1 -> ref_window_stop/1
  Constant12/1 -> rf_ref_chan_sel/1
  Register77/1 -> Register76/1
  Down Sample29/1 -> Register77/1
  Register76/1 -> rf_ref_amp/1
  Down Sample30/1 -> Register79/1
  Register79/1 -> Register78/1
  Register78/1 -> rf_ref_phase/1
  Register81/1 -> Register80/1
  Down Sample31/1 -> Register81/1
  Register80/1 -> rf_ref_i/1
  Down Sample32/1 -> Register83/1
  Register83/1 -> Register82/1
  Register82/1 -> rf_ref_q/1
  Register84/1 -> Up Sample8/1
  Register85/1 -> Register84/1
  Register87/1 -> Register86/1
  Register86/1 -> Up Sample9/1
  Register88/1 -> Up Sample10/1
  Register89/1 -> Register88/1
  rf_ref_amp/1 -> Terminator30/1
  rf_ref_phase/1 -> Terminator31/1
  rf_ref_i/1 -> Terminator32/1
  rf_ref_q/1 -> Terminator33/1
  In1/1 -> Bus Selector2/1
  Bus Selector2/1 -> Down Sample29/1  "<ref_amp>"
  Bus Selector2/2 -> Down Sample30/1  "<ref_phi>"
  Bus Selector2/3 -> Down Sample31/1  "<ref_i>"
  Bus Selector2/4 -> Down Sample32/1  "<ref_q>"
  Up Sample8/1 -> Bus Creator1/1  "ref_win_start"
  Up Sample9/1 -> Bus Creator1/2  "ref_win_stop"
  Up Sample10/1 -> Bus Creator1/3  "ref_chan_sel"
  Bus Creator1/1 -> Out1/1
  cav2_p1_if_i/1 -> Terminator41/1
  Register93/1 -> cav2_p1_amp_out/1
  Register91/1 -> cav2_p1_integrated_q/1
  cav2_p1_amp_out/1 -> Terminator36/1
  Register97/1 -> cav2_p1_if_amp/1
  cav2_p1_integrated_q/1 -> Terminator47/1
  Register96/1 -> cav2_p1_comparison_phase/1
  Register99/1 -> cav2_p1_if_i/1
  Register100/1 -> cav2_p1_if_q/1
  cav2_p1_dc_real/1 -> Terminator43/1
  cav2_p1_comparison_i/1 -> Terminator37/1
  Register90/1 -> cav2_p1_integrated_i/1
  Register94/1 -> cav2_p1_comparison_i/1
  Register92/1 -> cav2_p1_phase_out/1
  cav2_p1_dc_freq/1 -> Terminator45/1
  Register95/1 -> cav2_p1_comparison_q/1
  Register103/1 -> cav2_p1_dc_freq/1
  cav2_p1_integrated_i/1 -> Terminator46/1
  cav2_p1_comparison_phase/1 -> Terminator39/1
  cav2_p1_comparison_q/1 -> Terminator38/1
  cav2_p1_dc_img/1 -> Terminator44/1
  Register98/1 -> cav2_p1_if_phase/1
  Register101/1 -> cav2_p1_dc_real/1
  cav2_p1_if_amp/1 -> Terminator40/1
  cav2_p1_phase_out/1 -> Terminator35/1
  cav2_p1_if_phase/1 -> Terminator34/1
  Register102/1 -> cav2_p1_dc_img/1
  cav2_p1_if_q/1 -> Terminator42/1
  Down Sample33/1 -> Register104/1
  Register104/1 -> Register97/1
  Down Sample34/1 -> Register105/1
  Register105/1 -> Register98/1
  Down Sample35/1 -> Register106/1
  Register106/1 -> Register99/1
  Down Sample36/1 -> Register107/1
  Register107/1 -> Register100/1
  Down Sample37/1 -> Register108/1
  Register108/1 -> Register101/1
  Down Sample38/1 -> Register109/1
  Register109/1 -> Register102/1
  Down Sample39/1 -> Register110/1
  Register110/1 -> Register103/1
  Down Sample40/1 -> Register111/1
  Register111/1 -> Register90/1
  Down Sample41/1 -> Register112/1
  Register112/1 -> Register91/1
  Down Sample42/1 -> Register113/1
  Register113/1 -> Register92/1
  Down Sample43/1 -> Register114/1
  Register114/1 -> Register93/1
  Down Sample44/1 -> Register115/1
  Register115/1 -> Register94/1
  Down Sample45/1 -> Register116/1
  Register116/1 -> Register95/1
  Down Sample46/1 -> Register117/1
  Register117/1 -> Register96/1
  In4/1 -> Bus Selector3/1
  Bus Selector3/1 -> Down Sample33/1  "<c2p1_if_amp>"
  Bus Selector3/2 -> Down Sample34/1  "<c2p1_if_phi>"
  Bus Selector3/3 -> Down Sample35/1  "<c2p1_if_i>"
  Bus Selector3/4 -> Down Sample36/1  "<c2p1_if_q>"
  Bus Selector3/5 -> Down Sample37/1  "<c2p1_dc_i>"
  Bus Selector3/6 -> Down Sample38/1  "<c2p1_dc_q>"
  Bus Selector3/7 -> Down Sample39/1  "<c2p1_dc_freq>"
  Bus Selector3/8 -> Down Sample40/1  "<c2p1_integ_i>"
  Bus Selector3/9 -> Down Sample41/1  "<c2p1_integ_q>"
  Bus Selector3/10 -> Down Sample42/1  "<c2p1_phi_out>"
  Bus Selector3/11 -> Down Sample43/1  "<c2p1_amp_out>"
  Bus Selector3/12 -> Down Sample44/1  "<c2p1_comp_i>"
  Bus Selector3/13 -> Down Sample45/1  "<c2p1_comp_q>"
  Bus Selector3/14 -> Down Sample46/1  "<c2p1_comp_phi>"
  Register138/1 -> Register131/1
  Register144/1 -> Register123/1
  Register131/1 -> cav2_p2_dc_freq/1
  Register143/1 -> Register122/1
  Register130/1 -> cav2_p2_dc_img/1
  cav2_p2_dc_real/1 -> Terminator57/1
  Register124/1 -> cav2_p2_comparison_phase/1
  Register128/1 -> cav2_p2_if_q/1
  cav2_p2_integrated_q/1 -> Terminator61/1
  Register132/1 -> Register125/1
  "cav2_p2_if_i "/1 -> Terminator55/1
  cav2_p2_dc_img/1 -> Terminator58/1
  Register122/1 -> cav2_p2_comparison_i/1
  cav2_p2_phase_out/1 -> Terminator49/1
  Register141/1 -> Register120/1
  cav2_p2_if_phase/1 -> Terminator48/1
  Register140/1 -> Register119/1
  Register125/1 -> cav2_p2_if_amp/1
  Register127/1 -> "cav2_p2_if_i "/1
  Register145/1 -> Register124/1
  cav2_p2_if_q/1 -> Terminator56/1
  Register134/1 -> Register127/1
  cav2_p2_integrated_i/1 -> Terminator60/1
  Register126/1 -> cav2_p2_if_phase/1
  Register120/1 -> cav2_p2_phase_out/1
  Register121/1 -> cav2_p2_amp_out/1
  Register135/1 -> Register128/1
  Register137/1 -> Register130/1
  cav2_p2_if_amp/1 -> Terminator54/1
  cav2_p2_amp_out/1 -> Terminator50/1
  cav2_p2_comparison_i/1 -> Terminator51/1
  Register129/1 -> cav2_p2_dc_real/1
  Register118/1 -> cav2_p2_integrated_i/1
  cav2_p2_comparison_phase/1 -> Terminator53/1
  Register139/1 -> Register118/1
  Register142/1 -> Register121/1
  Register136/1 -> Register129/1
  cav2_p2_dc_freq/1 -> Terminator59/1
  cav2_p2_comparison_q/1 -> Terminator52/1
  Register123/1 -> cav2_p2_comparison_q/1
  Register133/1 -> Register126/1
  Register119/1 -> cav2_p2_integrated_q/1
  Down Sample47/1 -> Register132/1
  Down Sample48/1 -> Register133/1
  Down Sample49/1 -> Register134/1
  Down Sample50/1 -> Register135/1
  Down Sample51/1 -> Register136/1
  Down Sample52/1 -> Register137/1
  Down Sample53/1 -> Register138/1
  Down Sample54/1 -> Register139/1
  Down Sample55/1 -> Register140/1
  Down Sample56/1 -> Register141/1
  Down Sample57/1 -> Register142/1
  Down Sample58/1 -> Register143/1
  Down Sample59/1 -> Register144/1
  Down Sample60/1 -> Register145/1
  In5/1 -> Bus Selector4/1
  Bus Selector4/1 -> Down Sample47/1  "<c2p2_if_amp>"
  Bus Selector4/2 -> Down Sample48/1  "<c2p2_if_phi>"
  Bus Selector4/3 -> Down Sample49/1  "<c2p2_if_i>"
  Bus Selector4/4 -> Down Sample50/1  "<c2p2_if_q>"
  Bus Selector4/5 -> Down Sample51/1  "<c2p2_dc_i>"
  Bus Selector4/6 -> Down Sample52/1  "<c2p2_dc_q>"
  Bus Selector4/7 -> Down Sample53/1  "<c2p2_dc_freq>"
  Bus Selector4/8 -> Down Sample54/1  "<c2p2_integ_i>"
  Bus Selector4/9 -> Down Sample55/1  "<c2p2_integ_q>"
  Bus Selector4/10 -> Down Sample56/1  "<c2p2_phi_out>"
  Bus Selector4/11 -> Down Sample57/1  "<c2p2_amp_out>"
  Bus Selector4/12 -> Down Sample58/1  "<c2p2_comp_i>"
  Bus Selector4/13 -> Down Sample59/1  "<c2p2_comp_q>"
  Bus Selector4/14 -> Down Sample60/1  "<c2p2_comp_phi>"
  Constant6/1 -> cav2_p2_window_start/1, cav2_p1_window_start/1
  Constant11/1 -> Manual Switch3/1
  cav2_nco_phase_adj/1 -> Register161/1
  cav2_p2_window_stop/1 -> Register157/1
  cav2_nco_phase_reset/1 -> Register159/1
  Constant16/1 -> cav2_p1_chan_sel/1
  Repeating Sequence Stair1/1 -> Manual Switch1/1
  cav2_p1_window_stop/1 -> Register153/1
  cav2_p2_window_start/1 -> Register155/1
  cav2_p1_chan_sel/1 -> Register147/1
  cav2_p1_window_start/1 -> Register151/1
  Constant8/1 -> Manual Switch1/2
  Constant14/1 -> Manual Switch3/2
  Constant7/1 -> cav2_p2_window_stop/1, cav2_p1_window_stop/1
  Manual Switch1/1 -> cav2_nco_phase_adj/1
  cav2_p2_chan_sel/1 -> Register149/1
  Manual Switch3/1 -> cav2_nco_phase_reset/1
  Register147/1 -> Register146/1
  Register146/1 -> Up Sample11/1
  Register148/1 -> Up Sample12/1
  Register149/1 -> Register148/1
  Register151/1 -> Register150/1
  Register150/1 -> Up Sample13/1
  Register152/1 -> Up Sample14/1
  Register153/1 -> Register152/1
  Register155/1 -> Register154/1
  Register154/1 -> Up Sample15/1
  Register156/1 -> Up Sample16/1
  Register157/1 -> Register156/1
  Register159/1 -> Register158/1
  Register158/1 -> Up Sample17/1
  Register160/1 -> Up Sample18/1
  Register161/1 -> Register160/1
  Constant18/1 -> cav2_p2_chan_sel/1
  Up Sample11/1 -> Bus Creator2/1  "c2p1_chan_sel"
  Up Sample12/1 -> Bus Creator2/2  "c2p2_chan_sel"
  Up Sample13/1 -> Bus Creator2/3  "c2p1_win_start"
  Up Sample14/1 -> Bus Creator2/4  "c2p1_win_stop"
  Up Sample15/1 -> Bus Creator2/5  "c2p2_win_start"
  Up Sample16/1 -> Bus Creator2/6  "c2p2_win_stop"
  Up Sample17/1 -> Bus Creator2/7  "c2_nco_reset"
  Bus Creator2/1 -> Out3/1
  Register38/1 -> Terminator62/1
  Up Sample38/1 -> Bus Creator/8  "c1p1_cal_coeff"
  Register199/1 -> Register198/1
  Register198/1 -> Up Sample38/1
  cav1_p1_calibration_coeff/1 -> Register199/1
  Constant1/1 -> cav1_p1_calibration_coeff/1
  Constant2/1 -> cav1_p2_calibration_coeff/1
  cav1_p2_calibration_coeff/1 -> Register201/1
  Register200/1 -> Up Sample39/1
  Register201/1 -> Register200/1
  Up Sample39/1 -> Bus Creator/9  "c1p2_cal_coeff"
  Up Sample18/1 -> Bus Creator2/10  "c2_nco_phi"
  Register202/1 -> Up Sample40/1
  Up Sample41/1 -> Bus Creator2/9  "c2p2_cal_coeff"
  Register205/1 -> Register204/1
  Register203/1 -> Register202/1
  cav2_p2_calibration_coeff/1 -> Register205/1
  cav2_p1_calibration_coeff/1 -> Register203/1
  Constant21/1 -> cav2_p2_calibration_coeff/1
  Register204/1 -> Up Sample41/1
  Constant19/1 -> cav2_p1_calibration_coeff/1
  Up Sample40/1 -> Bus Creator2/8  "c2p1_cal_coeff"
